simulink model "feedback_simulation_2"  (R2023b)
settings: Solver=ode45  StartTime=0.0  StopTime=tc  MaxStep=1e-4  MinStep=1e-5  RelTol=1e-3
values from neighbouring files (symbols this model uses):
  d_a = 0    [lab5q2.m]
  d_y = 0    [lab5q2.m]
  rho = 1    [lab5q2.m]
libraries: cstblocks x2
settings Model: Creator=netcamo  LastModifiedBy=piercest
settings SolverCC: InitialStep=1e-5  AlgebraicLoopSolver=TrustRegion
settings DebuggingCC: UnconnectedInputMsg=warning  UnconnectedOutputMsg=warning  UnconnectedLineMsg=warning
settings ModelReferenceCC: EnableRefExpFcnMdlSchedulingChecks=on
settings RTWCC: DLArmComputeVersion=19.05

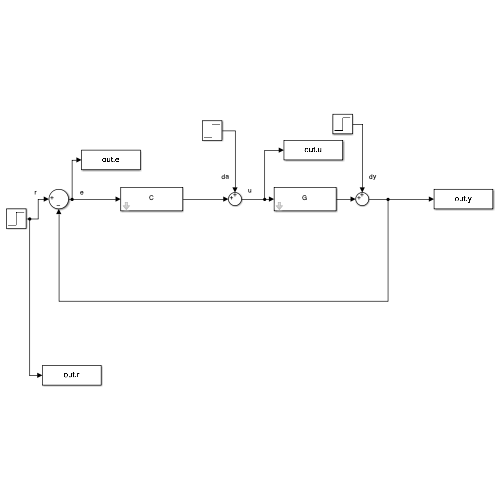
[thumbnail: Simulink's stored preview of the top-level diagram]
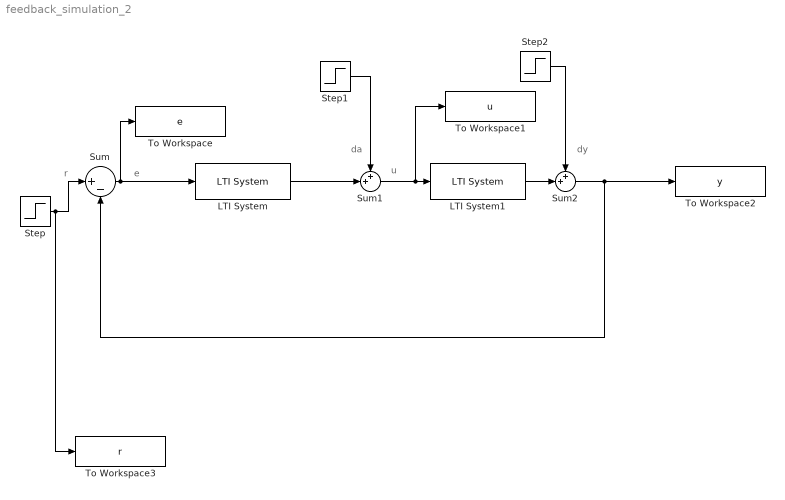
== system feedback_simulation_2 ==
  note: dy
  note: u
  note: da
  note: e
  note: r
  LTI System : cstblocks/LTI System  sys=C  IC=[]  PadeOrder=0
  LTI System1 : cstblocks/LTI System  sys=G  IC=[]  PadeOrder=0
  Step : Step  Time=0  After=rho  SampleTime=0
  Step1 : Step  Time=0  After=d_a  SampleTime=0
  Step2 : Step  Time=0  After=d_y  SampleTime=0
  Sum : Sum  Inputs=|+-
  Sum1 : Sum  Inputs=++|
  Sum2 : Sum  Inputs=++|
  To Workspace : ToWorkspace  VariableName=e  SaveFormat=Timeseries  SampleTime=-1
  To Workspace1 : ToWorkspace  VariableName=u  SaveFormat=Timeseries  SampleTime=-1
  To Workspace2 : ToWorkspace  VariableName=y  SaveFormat=Timeseries  SampleTime=-1
  To Workspace3 : ToWorkspace  VariableName=r  SaveFormat=Timeseries  SampleTime=-1
  wires:
  Step/1 -> To Workspace3/1, Sum/1
  Sum2/1 -> To Workspace2/1, Sum/2
  Sum/1 -> To Workspace/1, LTI System/1
  LTI System/1 -> Sum1/2
  Step1/1 -> Sum1/1
  Sum1/1 -> To Workspace1/1, LTI System1/1
  LTI System1/1 -> Sum2/2
  Step2/1 -> Sum2/1
